simulink model "lab_2_MC_integration"  (Simulink 7.3)
settings: Solver=ode3  StartTime=0.0  StopTime=100.0  FixedStep=1  RelTol=1e-3
undefined symbols (not defined in the file or in its folder): DiscIntNeverNeededParam
settings Model: Creator=IEUser  LastModifiedBy=IEUser
settings OptimizationCC: BooleanDataType=off

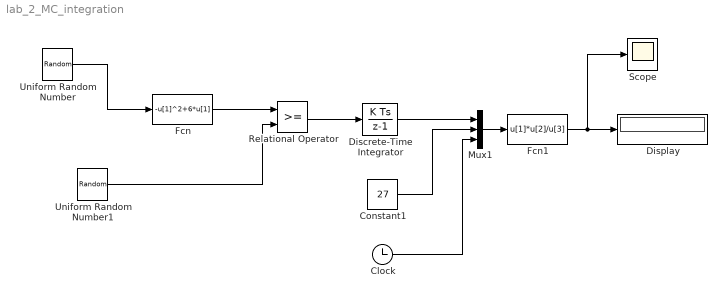
== system lab_2_MC_integration ==
  Clock : Clock
      settings: Decimation=10
  Constant1 : Constant  Value=27  OutDataType=fixdt(1, 16)  OutScaling=2^0
  Discrete-Time Integrator : DiscreteIntegrator  OutDataTypeMode=double  OutDataType=fixdt(1, 16)  OutScaling=2^0  OutDataTypeStr=double  ICPrevOutput=DiscIntNeverNeededParam  ICPrevScaledInput=DiscIntNeverNeededParam
  Display : Display
  Fcn : Fcn  Expr=-u[1]^2+6*u[1]
  Fcn1 : Fcn  Expr=u[1]*u[2]/u[3]
  Mux1 : Mux  Inputs=3
  Relational Operator : RelationalOperator  LogicOutDataTypeMode=boolean  LogicDataType=fixdt(0, 8)  OutDataTypeStr=boolean
  Scope : Scope
      settings: YMin=0  YMax=105
  Uniform Random Number : UniformRandomNumber  Minimum=2  Maximum=5  Seed=5  SampleTime=0
  Uniform Random Number1 : UniformRandomNumber  Minimum=0  Maximum=9  SampleTime=0
  wires:
  Fcn/1 -> Relational Operator/1
  Relational Operator/1 -> Discrete-Time Integrator/1
  Discrete-Time Integrator/1 -> Mux1/1
  Constant1/1 -> Mux1/2
  Clock/1 -> Mux1/3
  Mux1/1 -> Fcn1/1
  Fcn1/1 -> Display/1, Scope/1
  Uniform Random Number/1 -> Fcn/1
  Uniform Random Number1/1 -> Relational Operator/2
